simulink model "gm_sampleModel1899_sub"  (R2023a)
settings: Solver=VariableStepAuto  StartTime=0.0  StopTime=10.0  RelTol=1e-3
libraries: hdlsllib x6
settings Model: Creator=user1  LastModifiedBy=user1
settings OptimizationCC: BlockReduction=off  ConditionallyExecuteInputs=off
settings DebuggingCC: InheritedTsInSrcMsg=none

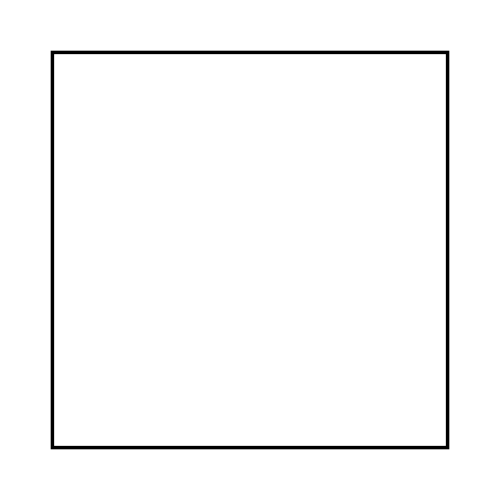
[thumbnail: Simulink's stored preview of the top-level diagram]
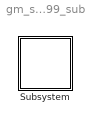
== system gm_sampleModel1899_sub ==
  Subsystem : Subsystem

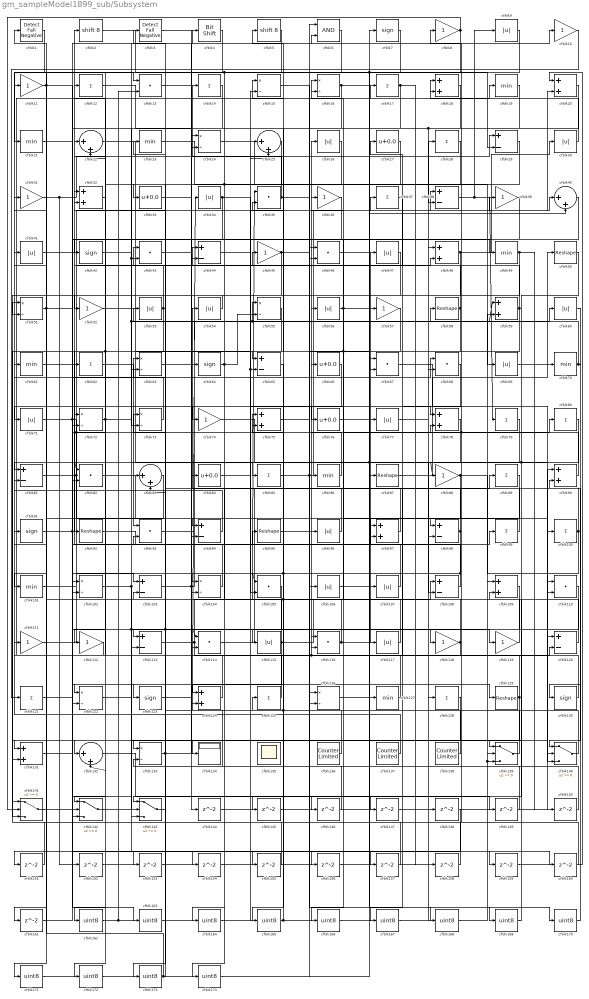
== system gm_sampleModel1899_sub/Subsystem ==
  cfblk1 : hdlsllib/Logic and Bit Operations/Detect Fall Negative  vinit=0  OutDataTypeStr=uint8
  cfblk{8,10..11,31,36,39,45,52,57,74,88,111..112,118..119} (15 alike) : Gain  OutDataTypeStr=uint8
  cfblk{12,14,17,28,37,62,79..80,85,89,99..100,121,125,128} (15 alike) : Sum  Inputs=+  OutDataTypeStr=uint8
  cfblk{19,21,23,49,61,70,86,101,127} (9 alike) : MinMax  OutDataTypeStr=uint8
  cfblk{15..16,24,51,55,63,72..73,102,104,122,126,133} (13 alike) : Product  Inputs=*/  OutDataTypeStr=uint8  RndMeth=Zero  SaturateOnIntegerOverflow=on
  cfblk{29,38,44,65,81,94,98,103,108,113,120} (11 alike) : Sum  Inputs=+-  OutDataTypeStr=uint8
  cfblk{13,35,43,46,67..68,82,93,105,110,114,116} (12 alike) : DotProduct  OutDataTypeStr=uint8
  cfblk{9,26,30,34,41,47,53..54,56,60,69,71,77,96,106..107,115,117} (18 alike) : Abs  OutDataTypeStr=uint8  SaturateOnIntegerOverflow=off
  cfblk{18,20,32,48,59,75,78,90,97,109,124,131} (12 alike) : Sum  OutDataTypeStr=uint8
  cfblk{7,42,64,91,123,130} (6 alike) : Signum
  cfblk{50,58,87,92,95,129} (6 alike) : Reshape
  cfblk{22,25,40,83,132} (5 alike) : Sum  Inputs=|++  OutDataTypeStr=uint8
  cfblk134 : Display
  cfblk135 : Scope
      settings: Floating=on
  cfblk136 : hdlsllib/Sources/Counter Limited  uplimit=7  tsamp=-1
  cfblk137 : hdlsllib/Sources/Counter Limited  uplimit=7  tsamp=-1
  cfblk138 : hdlsllib/Sources/Counter Limited  uplimit=7  tsamp=-1
  cfblk{139..143} (5 alike) : Switch  OutDataTypeStr=uint8  SaturateOnIntegerOverflow=off  InputSameDT=off
  cfblk{144..161} (18 alike) : Delay  SampleTime=1
  cfblk{162..174} (13 alike) : DataTypeConversion  OutDataTypeStr=uint8  SaturateOnIntegerOverflow=off  RndMeth=Floor
  cfblk2 : ArithShift  BitShiftNumber=8
  cfblk{27,33,66,76,84} (5 alike) : Bias  Bias=0.0  SaturateOnIntegerOverflow=off
  cfblk3 : hdlsllib/Logic and Bit Operations/Detect Fall Negative  vinit=0  OutDataTypeStr=uint8
  cfblk4 : hdlsllib/Logic and Bit Operations/Bit Shift  mode=Shift Left Logical  N=0
  cfblk5 : ArithShift  BitShiftNumber=8
  cfblk6 : Logic  AllPortsSameDT=off  OutDataTypeStr=boolean
  wires:
  cfblk174/1 -> cfblk57/1
  cfblk173/1 -> cfblk93/2, cfblk41/1
  cfblk172/1 -> cfblk46/2
  cfblk32/1 -> cfblk172/1
  cfblk171/1 -> cfblk46/1
  cfblk148/1 -> cfblk171/1
  cfblk170/1 -> cfblk90/2
  cfblk46/1 -> cfblk170/1
  cfblk169/1 -> cfblk109/2
  cfblk168/1 -> cfblk109/1
  cfblk76/1 -> cfblk168/1
  cfblk167/1 -> cfblk148/1
  cfblk109/1 -> cfblk167/1
  cfblk166/1 -> cfblk128/1
  cfblk165/1 -> cfblk139/3, cfblk139/2, cfblk125/1
  cfblk164/1 -> cfblk25/2
  cfblk163/1 -> cfblk25/1
  cfblk162/1 -> cfblk96/1, cfblk13/2
  cfblk161/1 -> cfblk72/2
  cfblk83/1 -> cfblk161/1
  cfblk160/1 -> cfblk18/2
  cfblk95/1 -> cfblk160/1
  cfblk159/1 -> cfblk20/1
  cfblk75/1 -> cfblk159/1
  cfblk158/1 -> cfblk141/1
  cfblk157/1 -> cfblk1/1
  cfblk15/1 -> cfblk157/1
  cfblk156/1 -> cfblk98/2
  cfblk131/1 -> cfblk156/1
  cfblk155/1 -> cfblk102/1
  cfblk122/1 -> cfblk155/1
  cfblk154/1 -> cfblk48/1
  cfblk153/1 -> cfblk103/2
  cfblk152/1 -> cfblk68/2
  cfblk151/1 -> cfblk51/1
  cfblk66/1 -> cfblk151/1
  cfblk150/1 -> cfblk126/1
  cfblk149/1 -> cfblk133/2
  cfblk132/1 -> cfblk149/1
  cfblk147/1 -> cfblk90/1
  cfblk37/1 -> cfblk147/1
  cfblk146/1 -> cfblk124/2
  cfblk145/1 -> cfblk6/1
  cfblk65/1 -> cfblk145/1
  cfblk144/1 -> cfblk59/2
  cfblk33/1 -> cfblk144/1
  cfblk129/1 -> cfblk141/3, cfblk87/1
  cfblk72/1 -> cfblk48/2, cfblk132/2
  cfblk1/1 -> cfblk11/1
  cfblk19/1 -> cfblk38/2, cfblk42/1
  cfblk100/1 -> cfblk53/1, cfblk140/3
  cfblk70/1 -> cfblk55/1, cfblk3/1, cfblk140/1
  cfblk82/1 -> cfblk94/1
  cfblk41/1 -> cfblk20/2
  cfblk14/1 -> cfblk73/2, cfblk43/2
  cfblk84/1 -> cfblk65/2, cfblk58/1
  cfblk68/1 -> cfblk97/1
  cfblk52/1 -> cfblk105/2
  cfblk102/1 -> cfblk114/1, cfblk140/2, cfblk59/1, cfblk19/1
  cfblk63/1 -> cfblk16/2
  cfblk108/1 -> cfblk105/1, cfblk12/1
  cfblk42/1 -> cfblk10/1
  cfblk130/1 -> cfblk72/1, cfblk116/1
  cfblk20/1 -> cfblk102/2
  cfblk40/1 -> cfblk132/1
  cfblk39/1 -> cfblk76/1
  cfblk24/1 -> cfblk106/1
  cfblk88/1 -> cfblk110/2, cfblk146/1
  cfblk110/1 -> cfblk113/2
  cfblk18/1 -> cfblk126/2
  cfblk106/1 -> cfblk127/1
  cfblk117/1 -> cfblk84/1
  cfblk16/1 -> cfblk88/1, cfblk119/1, cfblk65/1
  cfblk25/1 -> cfblk162/1
  cfblk126/1 -> cfblk107/1
  cfblk123/1 -> cfblk86/1
  cfblk136/1 -> cfblk45/1, cfblk83/2
  cfblk124/1 -> cfblk111/1
  cfblk99/1 -> cfblk32/1
  cfblk47/1 -> cfblk124/1
  cfblk26/1 -> cfblk133/1
  cfblk11/1 -> cfblk101/1, cfblk163/1
  cfblk74/1 -> cfblk100/1
  cfblk138/1 -> cfblk23/1
  cfblk121/1 -> cfblk95/1
  cfblk114/1 -> cfblk89/1
  cfblk67/1 -> cfblk120/1
  cfblk43/1 -> cfblk29/1
  cfblk3/1 -> cfblk129/1
  cfblk97/1 -> cfblk5/1
  cfblk143/1 -> cfblk73/1
  cfblk12/1 -> cfblk24/2
  cfblk94/1 -> cfblk81/2
  cfblk120/1 -> cfblk36/1
  cfblk96/1 -> cfblk62/1
  cfblk54/1 -> cfblk52/1
  cfblk78/1 -> cfblk108/2
  cfblk113/1 -> cfblk7/1, cfblk120/2
  cfblk13/1 -> cfblk104/2
  cfblk34/1 -> cfblk78/1, cfblk82/2
  cfblk87/1 -> cfblk50/1
  cfblk23/1 -> cfblk69/1
  cfblk45/1 -> cfblk104/1, cfblk67/2
  cfblk79/1 -> cfblk81/1
  cfblk44/1 -> cfblk15/2
  cfblk81/1 -> cfblk44/1, cfblk44/2, cfblk110/1
  cfblk6/1 -> cfblk74/1
  cfblk49/1 -> cfblk51/2, cfblk150/1
  cfblk28/1 -> cfblk33/1
  cfblk89/1 -> cfblk117/1
  cfblk61/1 -> cfblk37/1
  cfblk55/1 -> cfblk122/1, cfblk131/2
  cfblk5/1 -> cfblk131/1, cfblk174/1
  cfblk125/1 -> cfblk63/1
  cfblk9/1 -> cfblk112/1
  cfblk50/1 -> cfblk139/1
  cfblk141/1 -> cfblk4/1
  cfblk31/1 -> cfblk24/1, cfblk152/1
  cfblk69/1 -> cfblk70/1
  cfblk90/1 -> cfblk56/1, cfblk8/1
  cfblk119/1 -> cfblk35/2
  cfblk30/1 -> cfblk18/1
  cfblk56/1 -> cfblk16/1, cfblk40/1
  cfblk21/1 -> cfblk49/1
  cfblk91/1 -> cfblk64/1, cfblk118/1
  cfblk103/1 -> cfblk60/1, cfblk97/2
  cfblk142/1 -> cfblk77/1
  cfblk8/1 -> cfblk141/2, cfblk114/2
  cfblk62/1 -> cfblk93/1
  cfblk140/1 -> cfblk15/1
  cfblk51/1 -> cfblk31/1, cfblk143/3, cfblk71/1
  cfblk48/1 -> cfblk30/1, cfblk83/1
  cfblk77/1 -> cfblk28/1
  cfblk98/1 -> cfblk115/1, cfblk142/3, cfblk54/1
  cfblk2/1 -> cfblk67/1, cfblk29/2
  cfblk116/1 -> cfblk22/1, cfblk40/2
  cfblk127/1 -> cfblk66/1
  cfblk59/1 -> cfblk27/1, cfblk94/2
  cfblk36/1 -> cfblk142/1
  cfblk58/1 -> cfblk142/2, cfblk166/1, cfblk22/2
  cfblk107/1 -> cfblk47/1
  cfblk71/1 -> cfblk98/1, cfblk78/2
  cfblk53/1 -> cfblk92/1, cfblk32/2
  cfblk38/1 -> cfblk79/1, cfblk9/1
  cfblk60/1 -> cfblk130/1
  cfblk4/1 -> cfblk21/1
  cfblk133/1 -> cfblk43/1, cfblk6/2
  cfblk29/1 -> cfblk113/1
  cfblk115/1 -> cfblk108/1, cfblk91/1, cfblk122/2
  cfblk104/1 -> cfblk2/1
  cfblk22/1 -> cfblk85/1
  cfblk17/1 -> cfblk63/2, cfblk158/1
  cfblk7/1 -> cfblk134/1
  cfblk35/1 -> cfblk14/1, cfblk169/1
  cfblk85/1 -> cfblk38/1, cfblk39/1
  cfblk10/1 -> cfblk121/1
  cfblk73/1 -> cfblk61/1
  cfblk57/1 -> cfblk173/1
  cfblk105/1 -> cfblk143/2, cfblk153/1
  cfblk118/1 -> cfblk35/1, cfblk75/2, cfblk116/2
  cfblk86/1 -> cfblk26/1
  cfblk27/1 -> cfblk123/1, cfblk164/1
  cfblk137/1 -> cfblk13/1
  cfblk112/1 -> cfblk17/1
  cfblk139/1 -> cfblk34/1, cfblk75/1
  cfblk80/1 -> cfblk143/1, cfblk82/1
  cfblk101/1 -> cfblk103/1
  cfblk111/1 -> cfblk68/1
  cfblk128/1 -> cfblk165/1
  cfblk92/1 -> cfblk99/1
  cfblk93/1 -> cfblk80/1
  cfblk64/1 -> cfblk55/2, cfblk154/1
